simulink model "headingAlignment"  (R2019b)
settings: Solver=ode4  StartTime=tStart  StopTime=tEnd  FixedStep=tStep  RelTol=1e-3
values from neighbouring files (symbols this model uses):
  Heading_current_anim = headingCurrent    [simulation.m]
  headingCurrent = headings(ind)    [simulation.m]
  headingPrevious = -headingCurrent    [simulation.m]
  tStep = 0.1    [simulation.m]
  X = (1:imWidth)/imWidth*yardWidth    [getTerrainBinary1.m]
  XYPrevious = XYCurrent    [simulation.m]
  XYZ_current_anim = [XYPrevious(1) 0 XYPrevious(2)]    [simulation.m]
  Y = (1:imHeight)/imHeight*yardHeight    [getTerrainBinary1.m]
  Z = double(yardBright)/255*height    [createVirtualWorld.m]    (also in getTerrainBinary1.m = image; getTerrainBinary2.m = image; terrainMain.m = getTerrainBinary2(height, yardWidth, yardHeight, yardBright,)
libraries: simulink x1, vrlib x1
settings Model: Creator=sebas  LastModifiedBy=felixthomsen

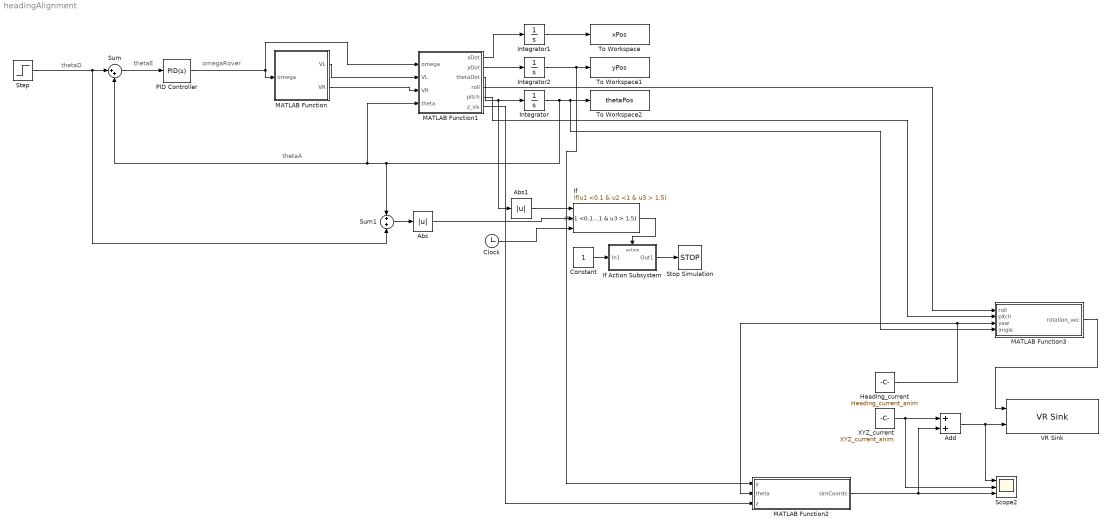
== system headingAlignment ==
  note: thetaD
  note: omegaRover
  note: thetaA
  note: thetaE
  Abs : Abs
  Abs1 : Abs
  Add : Sum
  Clock : Clock
  Constant : Constant
  "Heading_current " : Constant  Value=Heading_current_anim
  If : If  NumInputs=3  IfExpression=u1 <0.1 & u2 <1 & u3 > 1.5  ShowElse=off
  If Action Subsystem : Subsystem  TreatAsAtomicUnit=on
  Integrator : Integrator  InitialCondition=headingPrevious
  Integrator1 : Integrator
  Integrator2 : Integrator
  MATLAB Function : MATLAB Function  TreatAsAtomicUnit=on
  MATLAB Function1 : MATLAB Function  TreatAsAtomicUnit=on
  MATLAB Function2 : MATLAB Function  TreatAsAtomicUnit=on
  MATLAB Function3 : MATLAB Function  TreatAsAtomicUnit=on
  PID Controller : simulink/Continuous/PID Controller  Controller=PID  Form=Parallel  TimeDomain=Continuous-time  SampleTime=-1  IntegratorMethod=Forward Euler  FilterMethod=Forward Euler  ControllerParametersSource=internal  P=0.31  I=0.0004396  D=-0.0175  UseFilter=on  N=18.11  TunerSelectOption=Transfer Function Based (PID Tuner App)  InitialConditionSource=internal  InitialConditionForIntegrator=0  InitialConditionForFilter=0  DifferentiatorICPrevScaledInput=0  ExternalReset=none  TrackingMode=off  Kt=1  LimitOutput=off  UpperSaturationLimit=inf  LowerSaturationLimit=-inf  LinearizeAsGain=on  AntiWindupMode=none  Kb=1  POutMin=[]  POutMax=[]  IOutMin=[]  IOutMax=[]  DOutMin=[]  DOutMax=[]  NOutMin=[]  NOutMax=[]  SumOutMin=[]  SumOutMax=[]  SaturationOutMin=[]  SaturationOutMax=[]  PParamMin=[]  PParamMax=[]  IParamMin=[]  IParamMax=[]  DParamMin=[]  DParamMax=[]  NParamMin=[]  NParamMax=[]  KbParamMin=[]  KbParamMax=[]  KtParamMin=[]  KtParamMax=[]  KbOutMin=[]  KbOutMax=[]  KtOutMin=[]  KtOutMax=[]  IntegratorOutMin=[]  IntegratorOutMax=[]  FilterOutMin=[]  FilterOutMax=[]  SumI1OutMin=[]  SumI1OutMax=[]  SumI2OutMin=[]  SumI2OutMax=[]  SumI3OutMin=[]  SumI3OutMax=[]  SumI4OutMin=[]  SumI4OutMax=[]  SumDOutMin=[]  SumDOutMax=[]  DifferentiatorOutMin=[]  DifferentiatorOutMax=[]  FilterDiffOutCoefMin=[]  FilterDiffOutCoefMax=[]  ReciprocalOutMin=[]  ReciprocalOutMax=[]  SumDenOutMin=[]  SumDenOutMax=[]  SumNumOutMin=[]  SumNumOutMax=[]  DivideOutMin=[]  DivideOutMax=[]  IntegratorContinuousStateAttributes=''  IntegratorStateMustResolveToSignalObject=off  IntegratorRTWStateStorageClass=Auto  FilterContinuousStateAttributes=''  FilterStateMustResolveToSignalObject=off  FilterRTWStateStorageClass=Auto  ParallelPVariant=InternalParameters  IdealPVariant=Disabled  IVariant=InternalParameters  DVariant=InternalParameters  IntegratorVariant=Continuous  SatVariant=Disabled  AWVariant=Passthrough  PCopyVariant=Disabled  TRVariant=Disabled  FdbkBlocksVariant=Forward  IdealPFdbkVariant=Disabled  SatFdbkVariant=Disabled  DerivativeFilterVariant=ContFilter  NVariant=InternalParameters  NCopyVariant=Disabled  FilterICVariant=InternalICsFilter  IntegratorICVariant=InternalICs  ExternalResetVariant=Disabled  TRSumVariant=Passthrough  SumFdbkVariant=Disabled  SumVariant=Sum_PID
  Scope2 : Scope  NumInputPorts=3
  Step : Step  Time=0  Before=headingPrevious  After=headingCurrent  SampleTime=0
  Stop Simulation : Stop
  Sum : Sum  Inputs=|++
  Sum1 : Sum
  To Workspace : ToWorkspace  VariableName=xPos  SaveFormat=Timeseries  SampleTime=-1
  To Workspace1 : ToWorkspace  VariableName=yPos  SaveFormat=Timeseries  SampleTime=-1
  To Workspace2 : ToWorkspace  VariableName=thetaPos  SaveFormat=Timeseries  SampleTime=-1
  VR Sink : vrlib/VR Sink  InstantiateOnLoad=on  SampleTime=0.1  ViewEnable=on  RemoteChange=off  RemoteView=off  FieldsWritten=Rover_Transform.rotation.4.1.1.double#Rover_Transform.translation.3.1.1.double  WorldFileName=vrterrain_marsyardrover.wrl  AutoView=off  VideoDimensions=[]  AllowVariableSize=off
      settings: SourceProductName=Simulink
  "XYZ_current " : Constant  Value=XYZ_current_anim
  wires:
  Sum/1 -> PID Controller/1
  MATLAB Function1/1(xDot) -> Integrator1/1
  PID Controller/1 -> MATLAB Function1/1(omega), MATLAB Function/1(omega)
  MATLAB Function1/3(thetaDot) -> Abs1/1, Integrator/1
  MATLAB Function1/2(yDot) -> Integrator2/1
  Integrator1/1 -> To Workspace/1
  MATLAB Function/1(VL) -> MATLAB Function1/2(VL)
  MATLAB Function/2(VR) -> MATLAB Function1/3(VR)
  Step/1 -> Sum/1, Sum1/2
  Sum1/1 -> Abs/1
  Abs/1 -> If/2
  Abs1/1 -> If/1
  If Action Subsystem/1(Out1) -> Stop Simulation/1
  If/1 -> If Action Subsystem/Action
  Constant/1 -> If Action Subsystem/1(In1)
  Clock/1 -> If/3
  MATLAB Function1/6(z_vis) -> MATLAB Function2/3(z)
  MATLAB Function1/4(roll) -> MATLAB Function3/1(roll)
  MATLAB Function3/1(rotation_vec) -> VR Sink/1
  "Heading_current "/1 -> MATLAB Function3/3(yaw), MATLAB Function2/2(theta)
  MATLAB Function1/5(pitch) -> MATLAB Function3/2(pitch)
  Add/1 -> Scope2/1, VR Sink/2
  Integrator2/1 -> MATLAB Function2/1(y), To Workspace1/1
  "XYZ_current "/1 -> Scope2/2, Add/1
  MATLAB Function2/1(simCoords) -> Scope2/3, Add/2
  Integrator/1 -> MATLAB Function1/4(theta), Sum/2, Sum1/1, MATLAB Function3/4(angle), To Workspace2/1

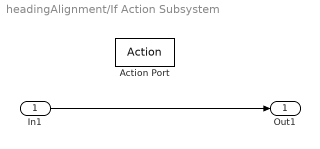
== system headingAlignment/If Action Subsystem ==
  In1 : Inport
  Action Port : ActionPort  ActionPortLabel=if(u1 <0.1 & u2 <1 & u3 > 1.5)
  Out1 : Outport
  wires:
  In1/1 -> Out1/1

== matlab function headingAlignment/MATLAB Function1 ==
  data: omega input; VL input; xDot output; VR input; yDot output; thetaDot output; XYPrevious parameter; X parameter; Y parameter; Z parameter; theta input; tStep parameter; roll output; pitch output; z_vis output
function [xDot,yDot,thetaDot, roll, pitch, z_vis] = kinematical(omega, VL, VR, XYPrevious, X, Y, Z, theta, tStep)


    n    = 4;                % number of wheels    (i)
    D    = 0.2286;           % diameter            (m)
    R    = D/2;              % radius              (m)
    lata = 0.5461;           % length axle to axle (m)
    wata = lata;             % width axle to axle  (m)
    ba   = [1, -1, -1, 1];   % x-wise position     (i)
    bb   = [1, 1, -1, -1];   % y-wise position     (i)

    headingNew = -theta+omega*tStep;
    headingOld = -theta;
%     pause(0.1)

    % convert straight line distance covered to updated xyz
    dcm1 = [cos(-headingNew) -sin(-headingNew);
        sin(-headingNew) cos(-headingNew)];
    wheel1True = [XYPrevious(1); XYPrevious(2)] + dcm1*[wata/2;lata/2];
    wheel2True = [XYPrevious(1); XYPrevious(2)] + dcm1*[-wata/2;lata/2];
    wheel3True = [XYPrevious(1); XYPrevious(2)] + dcm1*[-wata/2;-lata/2];
    wheel4True = [XYPrevious(1); XYPrevious(2)] + dcm1*[wata/2;-lata/2];
    wheelListXY = [wheel1True';wheel2True';wheel3True';wheel4True'];
    wheelXYZ = getWaypointsElevation(wheelListXY, X, Y, Z);

    
    dcm2 = [cos(-headingOld) -sin(-headingOld);
        sin(-headingOld) cos(-headingOld)];    
    wheel1TruePrev = [XYPrevious(1); XYPrevious(2)] + dcm2*[wata/2;lata/2];
    wheel2TruePrev = [XYPrevious(1); XYPrevious(2)] + dcm2*[-wata/2;lata/2];
    wheel3TruePrev = [XYPrevious(1); XYPrevious(2)] + dcm2*[-wata/2;-lata/2];
    wheel4TruePrev = [XYPrevious(1); XYPrevious(2)] + dcm2*[wata/2;-lata/2];
    wheelListXYPrev = [wheel1TruePrev';wheel2TruePrev';wheel3TruePrev';wheel4TruePrev'];
    wheelXYZPrev = getWaypointsElevation(wheelListXYPrev, X, Y, Z);
    
    
    bottom = sqrt((wheelXYZ(1,1)-wheelXYZPrev(1,1))^2 + (wheelXYZ(1,2)-wheelXYZPrev(1,2))^2);
    slope = atand((wheelXYZ(1,3)-wheelXYZPrev(1,3))/bottom);
    if isnan(slope) == 1
        wheel1Slope = 0;
    else
        wheel1Slope=slope;
    end
    
    bottom = sqrt((wheelXYZ(2,1)-wheelXYZPrev(2,1))^2 + (wheelXYZ(2,2)-wheelXYZPrev(2,2))^2);
    slope = atand((wheelXYZ(2,3)-wheelXYZPrev(2,3))/bottom);
    if isnan(slope) == 1
        wheel2Slope = 0;
    else
        wheel2Slope=slope;
    end
    
    bottom = sqrt((wheelXYZ(3,1)-wheelXYZPrev(3,1))^2 + (wheelXYZ(3,2)-wheelXYZPrev(3,2))^2);
    slope = atand((wheelXYZ(3,3)-wheelXYZPrev(3,3))/bottom);
    if isnan(slope) == 1
        wheel3Slope = 0;
    else
        wheel3Slope=slope;
    end
    
    bottom = sqrt((wheelXYZ(4,1)-wheelXYZPrev(4,1))^2 + (wheelXYZ(4,2)-wheelXYZPrev(4,2))^2);
    slope = atand((wheelXYZ(4,3)-wheelXYZPrev(4,3))/bottom);
    if isnan(slope) == 1
        wheel4Slope = 0;
    else
        wheel4Slope=slope;
    end  

    
    
    
        omega = [
        VR/abs(cosd(wheel1Slope));
        VL/abs(cosd(wheel2Slope));
        VL/abs(cosd(wheel3Slope));
        VR/abs(cosd(wheel4Slope))
        ]/R;

    
    
%     axis([-1 5 -1 5 -0.4 0.4])
%     plot3(wheelXYZ(:,1),wheelXYZ(:,2),wheelXYZ(:,3), 'Linewidth', 3)
%     hold off
    
%     omega = [VR;VL;VL;VR]/R;
    % HOMOGENOUS dimensions
    la = wata/2;    % reference to axle (X)
    lb = lata/2;    % reference to axle (Y)
    lc = la;        % reference to axle (Z)
    
    % WHEEL JACOBIAN (3 x 4)
    J    = (R/4)*[
            -1, 1, -1, 1; 
            1, 1, 1, 1; 
            1/(la + lb), -1/(la + lb), -1/(la + lb), 1/(la + lb)
        ];   

    rates = J*omega;
    xDot = rates(1);
    yDot = rates(2);
    thetaDot = rates(3);
    
    %return roll, pitch and z for visualisation - FELIX
    roll=atan((((wheelXYZ(2,3)+wheelXYZ(3,3))/2 - (wheelXYZ(1,3)+wheelXYZ(4,3))/2)/lata));
    pitch=atan((((wheelXYZ(2,3)+wheelXYZ(1,3))/2 - (wheelXYZ(2,3)+wheelXYZ(1,3))/2)/lata));

    z_vis=(wheelXYZ(4,3)+wheelXYZ(3,3)+wheelXYZ(2,3)+wheelXYZ(1,3))/4;

== matlab function headingAlignment/MATLAB Function ==
  data: omega input; VL output; VR output
function [VL,VR] = wheelVel(omega)
    
    width=0.5461;
    V = omega*width/2;
    
    VL = V;
    VR = -V;
    
    
%%%%%%%%%%%%%% ASSUMES TURNING ON SPOT
%%%%%%%%%% LEFT AND RIGHT WHEEL VELOCITIES ARE CONSTRAINED TO BE EQUAL
%%%%%%%%%% THINK THIS ASSUMES CLOCKWISE ROTATION?????

== matlab function headingAlignment/MATLAB Function2 ==
  data: simCoords output; y input; theta input; z input
function simCoords = coord_convert(y,theta,z)
       
       simCoords=zeros(1,3);
    
       %y input is distance along the path 
       %theta input is current heading

       %x output is actually y
       x_sim=cosd(theta)*y;
       %z output is actually x
       z_sim=sind(theta)*y;
       
       % y output is actually z 
       y_sim=z;
       
       simCoords=[x_sim y_sim z_sim-1];

== matlab function headingAlignment/MATLAB Function3 ==
  data: roll input; rotation_vec output size=[1 4]; pitch input; yaw input; angle input double [-360..360]
function rotation_vec = RotationVec(roll, pitch, yaw, angle)

    rotation_vec=zeros(1,4);
    
    angle=angle*pi/180;
    
    %determine the rotation matrices
    %Y is actually Z, Z is X and X is Y
    
    %for roll
    %this one needs to incorporate -pi/2 flip + roll
    theta=-pi/2+roll; %in rads
    R_x=[1 0 0;
        0 cos(theta) -sin(theta);
        0 sin(theta) cos(theta)];
    
    %for yaw
    theta=yaw; %in rads
    R_y=[cos(theta+angle-pi/2) 0 sin(theta+angle-pi/2);
        0 1 0;
        -sin(theta+angle-pi/2) 0 cos(theta+angle-pi/2)];
    
    %for pitch
    theta=pitch; %in rads
    R_z=[cos(theta) -sin(theta) 0;
        sin(theta) cos(theta) 0;
        0 0 1];
    
    rotm=R_z*R_y*R_x;
    %convert to angle-axis representation
    rotation_vec = rotm2axang(rotm);
